simulink model "part2s"  (R2024b)
settings: Solver=ode15s  StartTime=0.0  StopTime=10.0  MaxStep=0.01  RelTol=1e-3
values from neighbouring files (symbols this model uses):
  czas_skok = 0    [part1.m]
  L = acker(A', C', poles)'    [part1.m]
  x0 = [0; 0]    [part1.m]
  x_hat_0 = [0.5; 0.5]    [part1.m]
undefined symbols (not defined in the file or in its folder): A, B, C
settings Model: Creator=Adam  LastModifiedBy=Adam

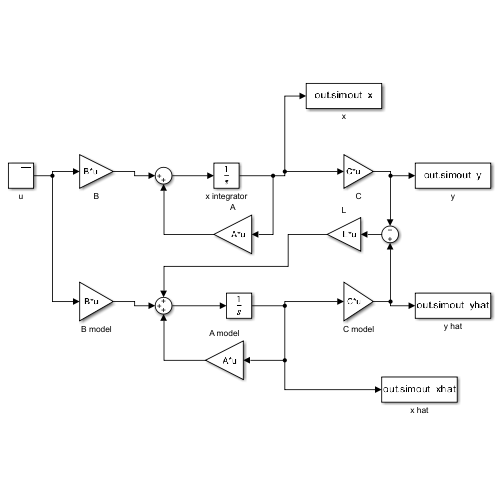
[thumbnail: Simulink's stored preview of the top-level diagram]
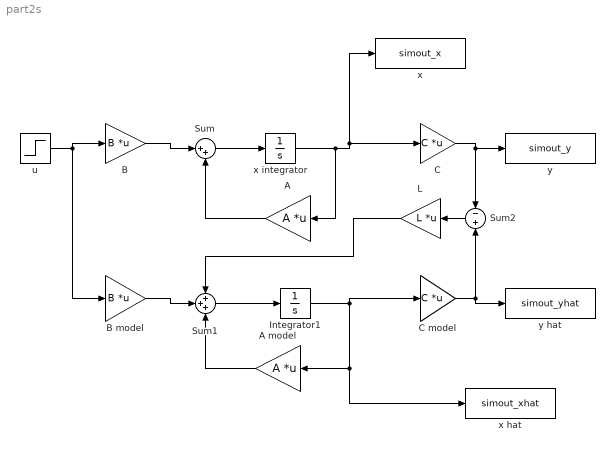
== system part2s ==
  A : Gain  Gain=A  Multiplication=Matrix(K*u)
  A model : Gain  Gain=A  Multiplication=Matrix(K*u)
  B : Gain  Gain=B  Multiplication=Matrix(K*u)
  B model : Gain  Gain=B  Multiplication=Matrix(K*u)
  C : Gain  Gain=C  Multiplication=Matrix(K*u)
  C model : Gain  Gain=C  Multiplication=Matrix(K*u)
  Integrator1 : Integrator  InitialCondition=x_hat_0
  L : Gain  Gain=L  Multiplication=Matrix(K*u)
  Sum : Sum  Inputs=|++
  Sum1 : Sum  Inputs=+++
  Sum2 : Sum  Inputs=-+
  u : Step  Time=czas_skok  SampleTime=0
  x : ToWorkspace  VariableName=simout_x  SampleTime=-1
  x hat : ToWorkspace  VariableName=simout_xhat  SampleTime=-1
  x integrator : Integrator  InitialCondition=x0
  y : ToWorkspace  VariableName=simout_y  SampleTime=-1
  y hat : ToWorkspace  VariableName=simout_yhat  SampleTime=-1
  wires:
  u/1 -> B model/1, B/1
  B/1 -> Sum/1
  C/1 -> Sum2/1, y/1
  Sum/1 -> x integrator/1
  x integrator/1 -> x/1, C/1, A/1
  A/1 -> Sum/2
  C model/1 -> y hat/1, Sum2/2
  Integrator1/1 -> x hat/1, A model/1, C model/1
  B model/1 -> Sum1/2
  A model/1 -> Sum1/3
  Sum1/1 -> Integrator1/1
  L/1 -> Sum1/1
  Sum2/1 -> L/1
